simulink model "P4_car"  (R2023b)
settings: Solver=VariableStepAuto  StartTime=0.0  StopTime=201  RelTol=1e-3
values from neighbouring files (symbols this model uses):
  rps2rpm = 60/(2*pi())    [P4init.m]
  track_waypoints = [transpose(track_x), transpose(track_y)]    [genTrack.m]
undefined symbols (not defined in the file or in its folder): batData, carData, motorData
libraries: slpidlib x2
settings Model: Creator=dxego  LastModifiedBy=kami2

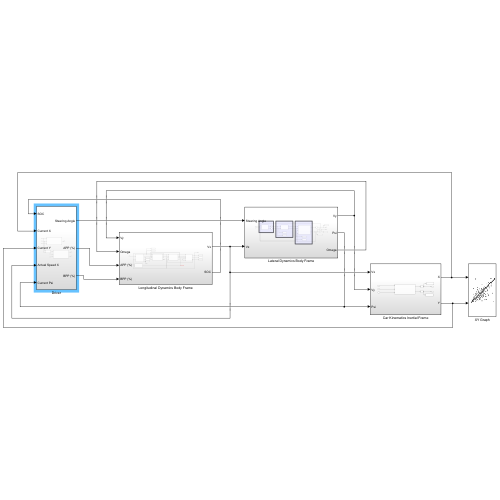
[thumbnail: Simulink's stored preview of the top-level diagram]
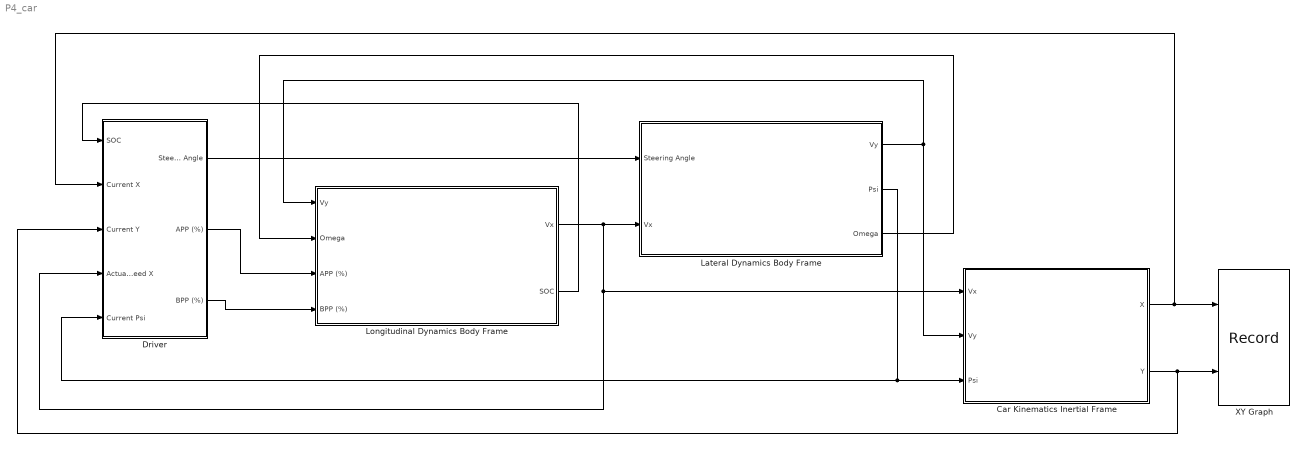
== system P4_car ==
  Car Kinematics Inertial Frame : Subsystem
  Driver : Subsystem
  Lateral Dynamics Body Frame : Subsystem
  Longitudinal Dynamics Body Frame : Subsystem
  XY Graph : Record  FileSettingsInternal="{\"entries\":[{\"content\":{\"excelSettings\":{\"content\":{},\"type\":\"Streamout.ExcelSettings\"}},\"type\":\"Streamout.FileSettingStorage\",\"uuid\":\"\"}],\"packageUris\":[\"http:\\/\\/schema.mathworks.com\\/mf0\\/streamout_blocks\\/R2020a\"],\"version\":\"1.0\"}"  Layout=[1 1]  SignalsInternal="{\"entries\":[{\"content\":{\"signals\":[{\"content\":{\"blockPath\":[],\"dimensions\":[1],\"domain\":\"\",\"lineColor\":\"#ff6929\",\"port\":1,\"sid\":[\"\"],\"signalID\":1460,\"signalName\":\"Car Kinematics Inertial Frame:1\"},\"type\":\"RecordBlkView.Signal\",\"uuid\":\"\"},{\"content\":{\"blockPath\":[],\"dimensions\":[1],\"domain\":\"\",\"lineColor\":\"#b746ff\",\"port\":2,\"sid\":[\"\"],\"signalID\":1464,\"signalName\":\"Car Kinematics Inertial Frame:2\"},\"type\":\"RecordBlkView.Signal\",\"uuid\":\"\"}]},\"type\":\"RecordBlkView.InputSignals\",\"uuid\":\"\"}],\"packageUris\":[\"http:\\/\\/schema.mathworks.com\\/mf0\\/streamout_blocks\\/R2020a\"],\"version\":\"1.0\"}"  VisualizationBindings="{\"xyplotplugin\":{\"info\":[{\"series\":[],\"subplotID\":1}]}}"  CompatibilityTag=XY  st=-1
  wires:
  Longitudinal Dynamics Body Frame/1(Vx) -> Driver/4(Actual Speed X), Car Kinematics Inertial Frame/1(Vx), Lateral Dynamics Body Frame/2(Vx)
  Lateral Dynamics Body Frame/1(Vy) -> Longitudinal Dynamics Body Frame/1(Vy), Car Kinematics Inertial Frame/2(Vy)
  Lateral Dynamics Body Frame/3(Omega) -> Longitudinal Dynamics Body Frame/2(Omega)
  Lateral Dynamics Body Frame/2(Psi) -> Car Kinematics Inertial Frame/3(Psi), Driver/5(Current Psi)
  Car Kinematics Inertial Frame/1(X) -> Driver/2(Current X), XY Graph/1
  Car Kinematics Inertial Frame/2(Y) -> XY Graph/2, Driver/3(Current Y)
  Driver/1(Steering Angle) -> Lateral Dynamics Body Frame/1(Steering Angle)
  Driver/2(APP (%)) -> Longitudinal Dynamics Body Frame/3(APP (%))
  Driver/3(BPP (%)) -> Longitudinal Dynamics Body Frame/4(BPP (%))
  Longitudinal Dynamics Body Frame/2(SOC) -> Driver/1(SOC)

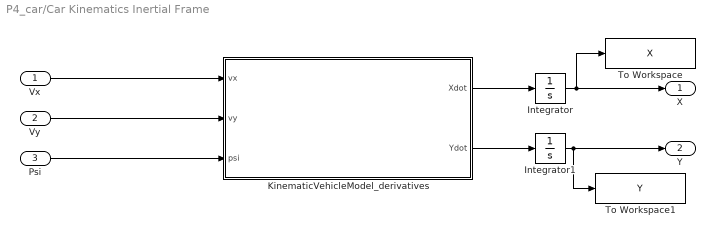
== system P4_car/Car Kinematics Inertial Frame ==
  Vx : Inport
  Vy : Inport  Port=2
  Psi : Inport  Port=3
  Integrator : Integrator  InitialCondition=carData.init.X0
  Integrator1 : Integrator  InitialCondition=carData.init.Y0
  KinematicVehicleModel_derivatives : MATLAB Function  TreatAsAtomicUnit=on  mask{obj=carData}
      mask prompts: obj "obj structure"
  To Workspace : ToWorkspace  VariableName=X  SaveFormat=Timeseries  SampleTime=-1
  To Workspace1 : ToWorkspace  VariableName=Y  SaveFormat=Timeseries  SampleTime=-1
  X : Outport
  Y : Outport  Port=2
  wires:
  KinematicVehicleModel_derivatives/1(Xdot) -> Integrator/1
  KinematicVehicleModel_derivatives/2(Ydot) -> Integrator1/1
  Integrator/1 -> To Workspace/1, X/1
  Integrator1/1 -> To Workspace1/1, Y/1
  Vx/1 -> KinematicVehicleModel_derivatives/1(vx)
  Vy/1 -> KinematicVehicleModel_derivatives/2(vy)
  Psi/1 -> KinematicVehicleModel_derivatives/3(psi)

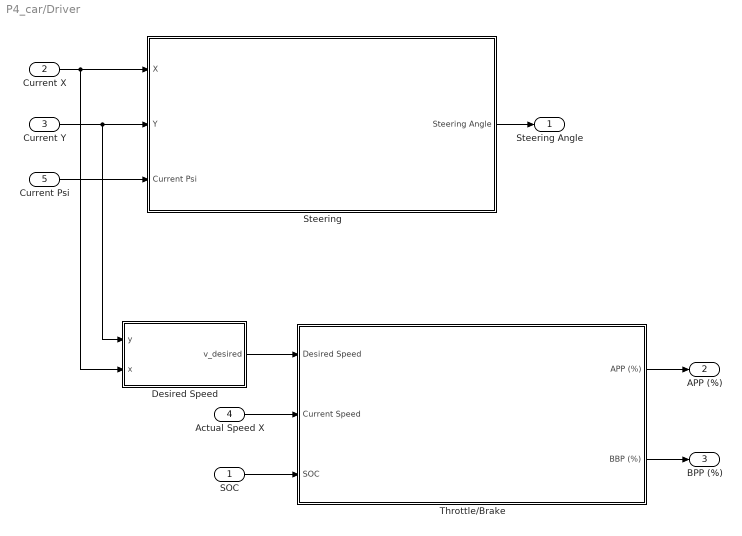
== system P4_car/Driver ==
  SOC : Inport
  Current X : Inport  Port=2
  Current Y : Inport  Port=3
  Actual Speed X : Inport  Port=4
  Current Psi : Inport  Port=5
  Desired Speed : MATLAB Function  TreatAsAtomicUnit=on
  Steering : Subsystem
  Throttle/Brake : Subsystem
  Steering Angle : Outport
  APP (%) : Outport  Port=2
  BPP (%) : Outport  Port=3
  wires:
  Current X/1 -> Desired Speed/2(x), Steering/1(X)
  Current Y/1 -> Steering/2(Y), Desired Speed/1(y)
  SOC/1 -> Throttle/Brake/3(SOC)
  Actual Speed X/1 -> Throttle/Brake/2(Current Speed)
  Throttle/Brake/1(APP (%)) -> APP (%)/1
  Throttle/Brake/2(BBP (%)) -> BPP (%)/1
  Steering/1(Steering Angle) -> Steering Angle/1
  Current Psi/1 -> Steering/3(Current Psi)
  Desired Speed/1(v_desired) -> Throttle/Brake/1(Desired Speed)

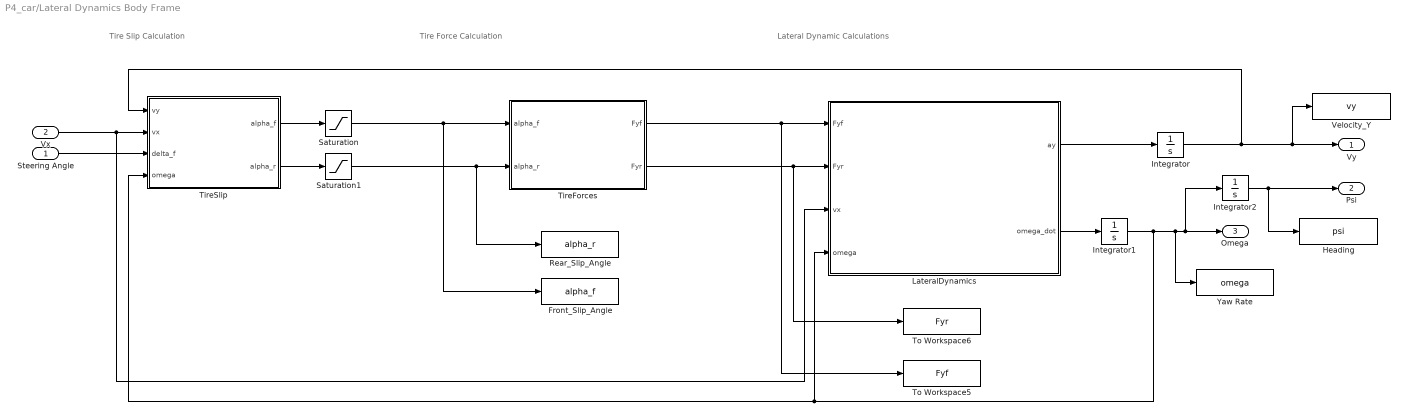
== system P4_car/Lateral Dynamics Body Frame ==
  note: Tire Slip Calculation
  note: Tire Force Calculation
  note: Lateral Dynamic Calculations
  Steering Angle : Inport
  Vx : Inport  Port=2
  Front_Slip_Angle : ToWorkspace  VariableName=alpha_f  SaveFormat=Timeseries  SampleTime=-1
  Heading : ToWorkspace  VariableName=psi  SaveFormat=Timeseries  SampleTime=-1
  Integrator : Integrator  InitialCondition=carData.init.vy0
  Integrator1 : Integrator  InitialCondition=carData.init.omega0
  Integrator2 : Integrator  InitialCondition=carData.init.psi0
  LateralDynamics : MATLAB Function  TreatAsAtomicUnit=on  mask{obj=carData}
      mask prompts: obj "obj structure"
  Rear_Slip_Angle : ToWorkspace  VariableName=alpha_r  SaveFormat=Timeseries  SampleTime=-1
  Saturation : Saturate  UpperLimit=carData.maxAlpha  LowerLimit=-carData.maxAlpha
  Saturation1 : Saturate  UpperLimit=carData.maxAlpha  LowerLimit=-carData.maxAlpha
  TireForces : MATLAB Function  TreatAsAtomicUnit=on  mask{obj=carData}
      mask prompts: obj "obj structure"
  TireSlip : MATLAB Function  TreatAsAtomicUnit=on  mask{obj=carData}
      mask prompts: obj "obj structure"
  To Workspace5 : ToWorkspace  VariableName=Fyf  SaveFormat=Timeseries  SampleTime=-1
  To Workspace6 : ToWorkspace  VariableName=Fyr  SaveFormat=Timeseries  SampleTime=-1
  Velocity_Y : ToWorkspace  VariableName=vy  SaveFormat=Timeseries  SampleTime=-1
  Yaw Rate : ToWorkspace  VariableName=omega  SaveFormat=Timeseries  SampleTime=-1
  Vy : Outport
  Psi : Outport  Port=2
  Omega : Outport  Port=3
  wires:
  LateralDynamics/1(ay) -> Integrator/1
  Integrator/1 -> Vy/1, Velocity_Y/1, TireSlip/1(vy)
  LateralDynamics/2(omega_dot) -> Integrator1/1
  Integrator1/1 -> Integrator2/1, Omega/1, Yaw Rate/1, LateralDynamics/4(omega), TireSlip/4(omega)
  TireSlip/1(alpha_f) -> Saturation/1
  TireSlip/2(alpha_r) -> Saturation1/1
  TireForces/1(Fyf) -> LateralDynamics/1(Fyf), To Workspace5/1
  TireForces/2(Fyr) -> LateralDynamics/2(Fyr), To Workspace6/1
  Saturation/1 -> TireForces/1(alpha_f), Front_Slip_Angle/1
  Saturation1/1 -> TireForces/2(alpha_r), Rear_Slip_Angle/1
  Vx/1 -> TireSlip/2(vx), LateralDynamics/3(vx)
  Steering Angle/1 -> TireSlip/3(delta_f)
  Integrator2/1 -> Heading/1, Psi/1

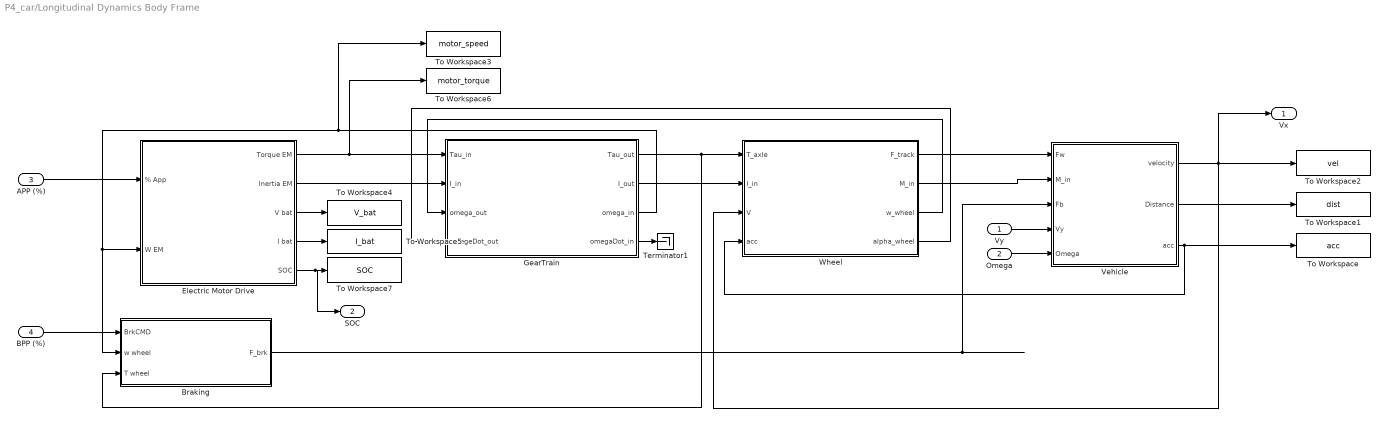
== system P4_car/Longitudinal Dynamics Body Frame ==
  Vy : Inport
  Omega : Inport  Port=2
  APP (%) : Inport  Port=3
  BPP (%) : Inport  Port=4
  Braking : Subsystem
  Electric Motor Drive : Subsystem
  GearTrain : Subsystem
  Terminator1 : Terminator
  To Workspace : ToWorkspace  VariableName=acc  SaveFormat=Timeseries  SampleTime=-1
  To Workspace1 : ToWorkspace  VariableName=dist  SaveFormat=Timeseries  SampleTime=-1
  To Workspace2 : ToWorkspace  VariableName=vel  SaveFormat=Timeseries  SampleTime=-1
  To Workspace3 : ToWorkspace  VariableName=motor_speed  SaveFormat=Timeseries  SampleTime=-1
  To Workspace4 : ToWorkspace  VariableName=V_bat  SaveFormat=Timeseries  SampleTime=-1
  To Workspace5 : ToWorkspace  VariableName=I_bat  SaveFormat=Timeseries  SampleTime=-1
  To Workspace6 : ToWorkspace  VariableName=motor_torque  SaveFormat=Timeseries  SampleTime=-1
  To Workspace7 : ToWorkspace  VariableName=SOC  SaveFormat=Timeseries  SampleTime=-1
  Vehicle : Subsystem
  "Wheel " : Subsystem
  Vx : Outport
  SOC : Outport  Port=2
  wires:
  "Wheel "/2(M_in) -> Vehicle/2("M_in ")
  Electric Motor Drive/2(Inertia EM) -> GearTrain/2(I_in)
  GearTrain/4(omegaDot_in) -> Terminator1/1
  Electric Motor Drive/3(V bat) -> To Workspace4/1
  Vehicle/2("Distance ") -> To Workspace1/1
  Electric Motor Drive/1(Torque EM) -> To Workspace6/1, GearTrain/1(Tau_in)
  Vehicle/3(acc) -> "Wheel "/4(acc), To Workspace/1
  Electric Motor Drive/4(I bat) -> To Workspace5/1
  "Wheel "/3(w_wheel) -> GearTrain/3(omega_out)
  GearTrain/3(omega_in) -> To Workspace3/1, Electric Motor Drive/2(W EM), Braking/2("w wheel ")
  Vehicle/1("velocity ") -> Vx/1, To Workspace2/1, "Wheel "/3(V)
  "Wheel "/4(alpha_wheel) -> GearTrain/4(omegeDot_out)
  Braking/1("F_brk ") -> Vehicle/3("Fb ")
  GearTrain/1(Tau_out) -> Braking/3(T wheel), "Wheel "/1(T_axle)
  "Wheel "/1(F_track) -> Vehicle/1("Fw ")
  GearTrain/2(I_out) -> "Wheel "/2(I_in)
  Electric Motor Drive/5(SOC) -> SOC/1, To Workspace7/1
  APP (%)/1 -> Electric Motor Drive/1(% App)
  BPP (%)/1 -> Braking/1("BrkCMD ")
  Vy/1 -> Vehicle/4(Vy)
  Omega/1 -> Vehicle/5(Omega)

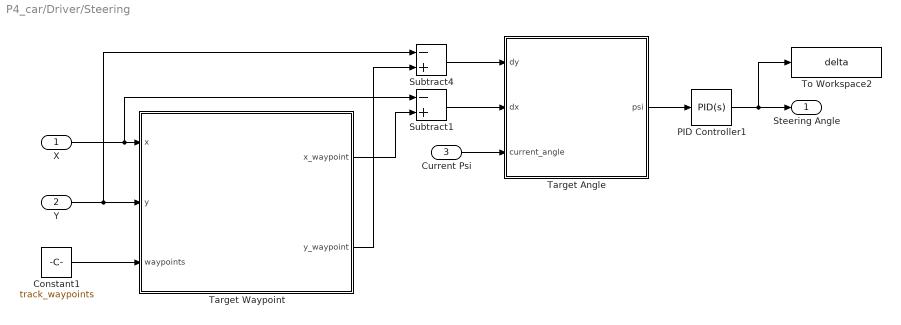
== system P4_car/Driver/Steering ==
  X : Inport
  Y : Inport  Port=2
  Current Psi : Inport  Port=3
  Constant1 : Constant  Value=track_waypoints
  PID Controller1 : slpidlib/PID Controller  Controller=PID  Form=Parallel  TimeDomain=Continuous-time  UseExternalTs=off  SampleTime=-1  IntegratorMethod=Forward Euler  FilterMethod=Forward Euler  ControllerParametersSource=internal  P=0.5  I=0  UseKiTs=off  D=0  N=100  UseFilter=on  TunerSelectOption=Transfer Function Based (PID Tuner App)  InitialConditionSource=internal  InitialConditionForIntegrator=0  InitialConditionForFilter=0  DifferentiatorICPrevScaledInput=0  ExternalReset=none  TrackingMode=off  Kt=1  LimitOutput=off  SatLimitsSource=internal  UpperSaturationLimit=inf  LowerSaturationLimit=-inf  LinearizeAsGain=on  AntiWindupMode=none  Kb=1  LimitIntegrator=off  UpperIntegratorSaturationLimit=inf  LowerIntegratorSaturationLimit=-inf  POutMin=[]  POutMax=[]  IOutMin=[]  IOutMax=[]  DOutMin=[]  DOutMax=[]  NOutMin=[]  NOutMax=[]  SumOutMin=[]  SumOutMax=[]  SaturationOutMin=[]  SaturationOutMax=[]  PParamMin=[]  PParamMax=[]  IParamMin=[]  IParamMax=[]  DParamMin=[]  DParamMax=[]  NParamMin=[]  NParamMax=[]  KbParamMin=[]  KbParamMax=[]  KtParamMin=[]  KtParamMax=[]  KbOutMin=[]  KbOutMax=[]  KtOutMin=[]  KtOutMax=[]  IntegratorOutMin=[]  IntegratorOutMax=[]  FilterOutMin=[]  FilterOutMax=[]  SumI1OutMin=[]  SumI1OutMax=[]  SumI2OutMin=[]  SumI2OutMax=[]  SumI3OutMin=[]  SumI3OutMax=[]  SumI4OutMin=[]  SumI4OutMax=[]  SumDOutMin=[]  SumDOutMax=[]  DifferentiatorOutMin=[]  DifferentiatorOutMax=[]  FilterDiffOutCoefMin=[]  FilterDiffOutCoefMax=[]  ReciprocalOutMin=[]  ReciprocalOutMax=[]  SumDenOutMin=[]  SumDenOutMax=[]  SumNumOutMin=[]  SumNumOutMax=[]  DivideOutMin=[]  DivideOutMax=[]  UdiffTsProdOutMin=[]  UdiffTsProdOutMax=[]  NTsProdOutMin=[]  NTsProdOutMax=[]  UintegralTsProdOutMin=[]  UintegralTsProdOutMax=[]  UngainTsProdOutMin=[]  UngainTsProdOutMax=[]  ClampingZeroOutDataTypeStr=Inherit: Inherit via back propagation  ClampingZeroOutMin=[]  ClampingZeroOutMax=[]  FilterDenConstantOutDataTypeStr=Inherit: Inherit via back propagation  FilterDenConstantOutMin=[]  FilterDenConstantOutMax=[]  PCopyOutDataTypeStr=Inherit: Inherit via back propagation  PCopyOutMin=[]  PCopyOutMax=[]  NCopyOutDataTypeStr=Inherit: Inherit via back propagation  NCopyOutMin=[]  NCopyOutMax=[]  IntegratorContinuousStateAttributes=''  IntegratorStateMustResolveToSignalObject=off  IntegratorRTWStateStorageClass=Auto  FilterContinuousStateAttributes=''  FilterStateMustResolveToSignalObject=off  FilterRTWStateStorageClass=Auto  ParallelPVariant=InternalParameters  IdealPVariant=Disabled  IVariant=InternalParameters  DVariant=InternalParameters  IntegratorVariant=Continuous  SatVariant=Disabled  AWVariant=Passthrough  PCopyVariant=Disabled  TRVariant=Disabled  FdbkBlocksVariant=Forward  IdealPFdbkVariant=Disabled  SatFdbkVariant=Disabled  DerivativeFilterVariant=ContFilter  NVariant=InternalParameters  NCopyVariant=Disabled  FilterICVariant=InternalICsFilter  IntegratorICVariant=InternalICs  ExternalResetVariant=Disabled  TRSumVariant=Passthrough  SumFdbkVariant=Disabled  SumVariant=Sum_PID  TsampFilterVariant=InternalTs  TsampNgainVariant=Passthrough  TsampIntegralVariant=Disabled_SignalSpec  ExternalSaturationOutDataTypeStr=Inherit: Same as second input
  Subtract1 : Sum  Inputs=-+
  Subtract4 : Sum  Inputs=-+
  Target Angle : MATLAB Function  TreatAsAtomicUnit=on
  Target Waypoint : MATLAB Function  TreatAsAtomicUnit=on
  To Workspace2 : ToWorkspace  VariableName=delta  SaveFormat=Timeseries  SampleTime=-1
  Steering Angle : Outport
  wires:
  Constant1/1 -> Target Waypoint/3(waypoints)
  Target Waypoint/2(y_waypoint) -> Subtract4/2
  Y/1 -> Subtract4/1, Target Waypoint/2(y)
  X/1 -> Target Waypoint/1(x), Subtract1/1
  Subtract1/1 -> Target Angle/2(dx)
  Target Angle/1(psi) -> PID Controller1/1
  Current Psi/1 -> Target Angle/3(current_angle)
  Target Waypoint/1(x_waypoint) -> Subtract1/2
  Subtract4/1 -> Target Angle/1(dy)
  PID Controller1/1 -> To Workspace2/1, Steering Angle/1

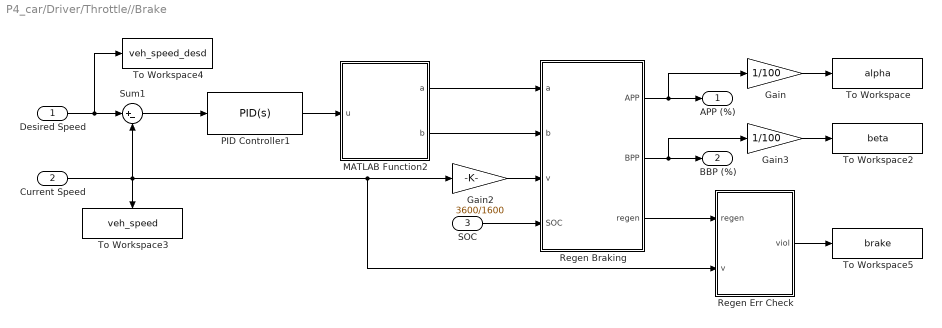
== system P4_car/Driver/Throttle//Brake ==
  Desired Speed : Inport
  Current Speed : Inport  Port=2
  SOC : Inport  Port=3
  Gain : Gain  Gain=1/100
  Gain2 : Gain  Gain=3600/1600
  Gain3 : Gain  Gain=1/100
  MATLAB Function2 : MATLAB Function  TreatAsAtomicUnit=on
  PID Controller1 : slpidlib/PID Controller  Controller=PID  Form=Parallel  TimeDomain=Continuous-time  UseExternalTs=off  SampleTime=-1  IntegratorMethod=Forward Euler  FilterMethod=Forward Euler  ControllerParametersSource=internal  P=.5  I=0  UseKiTs=off  D=0  N=100  UseFilter=on  TunerSelectOption=Transfer Function Based (PID Tuner App)  InitialConditionSource=internal  InitialConditionForIntegrator=0  InitialConditionForFilter=0  DifferentiatorICPrevScaledInput=0  ExternalReset=none  TrackingMode=off  Kt=1  LimitOutput=on  SatLimitsSource=internal  UpperSaturationLimit=1  LowerSaturationLimit=-1  LinearizeAsGain=off  AntiWindupMode=none  Kb=1  LimitIntegrator=off  UpperIntegratorSaturationLimit=inf  LowerIntegratorSaturationLimit=-inf  POutMin=[]  POutMax=[]  IOutMin=[]  IOutMax=[]  DOutMin=[]  DOutMax=[]  NOutMin=[]  NOutMax=[]  SumOutMin=[]  SumOutMax=[]  SaturationOutMin=[]  SaturationOutMax=[]  PParamMin=[]  PParamMax=[]  IParamMin=[]  IParamMax=[]  DParamMin=[]  DParamMax=[]  NParamMin=[]  NParamMax=[]  KbParamMin=[]  KbParamMax=[]  KtParamMin=[]  KtParamMax=[]  KbOutMin=[]  KbOutMax=[]  KtOutMin=[]  KtOutMax=[]  IntegratorOutMin=[]  IntegratorOutMax=[]  FilterOutMin=[]  FilterOutMax=[]  SumI1OutMin=[]  SumI1OutMax=[]  SumI2OutMin=[]  SumI2OutMax=[]  SumI3OutMin=[]  SumI3OutMax=[]  SumI4OutMin=[]  SumI4OutMax=[]  SumDOutMin=[]  SumDOutMax=[]  DifferentiatorOutMin=[]  DifferentiatorOutMax=[]  FilterDiffOutCoefMin=[]  FilterDiffOutCoefMax=[]  ReciprocalOutMin=[]  ReciprocalOutMax=[]  SumDenOutMin=[]  SumDenOutMax=[]  SumNumOutMin=[]  SumNumOutMax=[]  DivideOutMin=[]  DivideOutMax=[]  UdiffTsProdOutMin=[]  UdiffTsProdOutMax=[]  NTsProdOutMin=[]  NTsProdOutMax=[]  UintegralTsProdOutMin=[]  UintegralTsProdOutMax=[]  UngainTsProdOutMin=[]  UngainTsProdOutMax=[]  ClampingZeroOutDataTypeStr=Inherit: Inherit via back propagation  ClampingZeroOutMin=[]  ClampingZeroOutMax=[]  FilterDenConstantOutDataTypeStr=Inherit: Inherit via back propagation  FilterDenConstantOutMin=[]  FilterDenConstantOutMax=[]  PCopyOutDataTypeStr=Inherit: Inherit via back propagation  PCopyOutMin=[]  PCopyOutMax=[]  NCopyOutDataTypeStr=Inherit: Inherit via back propagation  NCopyOutMin=[]  NCopyOutMax=[]  IntegratorContinuousStateAttributes=''  IntegratorStateMustResolveToSignalObject=off  IntegratorRTWStateStorageClass=Auto  FilterContinuousStateAttributes=''  FilterStateMustResolveToSignalObject=off  FilterRTWStateStorageClass=Auto  ParallelPVariant=InternalParameters  IdealPVariant=Disabled  IVariant=InternalParameters  DVariant=InternalParameters  IntegratorVariant=Continuous  SatVariant=Enabled  AWVariant=Passthrough  PCopyVariant=Disabled  TRVariant=Disabled  FdbkBlocksVariant=Forward  IdealPFdbkVariant=Disabled  SatFdbkVariant=Disabled  DerivativeFilterVariant=ContFilter  NVariant=InternalParameters  NCopyVariant=Disabled  FilterICVariant=InternalICsFilter  IntegratorICVariant=InternalICs  ExternalResetVariant=Disabled  TRSumVariant=Passthrough  SumFdbkVariant=Disabled  SumVariant=Sum_PID  TsampFilterVariant=InternalTs  TsampNgainVariant=Passthrough  TsampIntegralVariant=Disabled_SignalSpec  ExternalSaturationOutDataTypeStr=Inherit: Same as second input
  Regen Braking : MATLAB Function  TreatAsAtomicUnit=on
  Regen Err Check : MATLAB Function  TreatAsAtomicUnit=on
  Sum1 : Sum  Inputs=|+-
  To Workspace : ToWorkspace  VariableName=alpha  SaveFormat=Timeseries  SampleTime=-1
  To Workspace2 : ToWorkspace  VariableName=beta  SaveFormat=Timeseries  SampleTime=-1
  To Workspace3 : ToWorkspace  VariableName=veh_speed  SaveFormat=Timeseries  SampleTime=-1
  To Workspace4 : ToWorkspace  VariableName=veh_speed_desd  SaveFormat=Timeseries  SampleTime=-1
  To Workspace5 : ToWorkspace  VariableName=brake  SaveFormat=Timeseries  SampleTime=-1
  APP (%) : Outport
  BBP (%) : Outport  Port=2
  wires:
  PID Controller1/1 -> MATLAB Function2/1(u)
  MATLAB Function2/2(b) -> Regen Braking/2(b)
  Regen Braking/3(regen) -> Regen Err Check/1(regen)
  Regen Braking/2(BPP) -> Gain3/1, BBP (%)/1
  Regen Err Check/1(viol) -> To Workspace5/1
  SOC/1 -> Regen Braking/4(SOC)
  Desired Speed/1 -> To Workspace4/1, Sum1/1
  MATLAB Function2/1(a) -> Regen Braking/1(a)
  Sum1/1 -> PID Controller1/1
  Current Speed/1 -> To Workspace3/1, Sum1/2, Regen Err Check/2(v), Gain2/1
  Gain2/1 -> Regen Braking/3(v)
  Regen Braking/1(APP) -> Gain/1, APP (%)/1
  Gain/1 -> To Workspace/1
  Gain3/1 -> To Workspace2/1

== system P4_car/Longitudinal Dynamics Body Frame/Braking ==
  "BrkCMD " : Inport
  "w wheel " : Inport  Port=2
  T wheel : Inport  Port=3
  Constant : Constant  Value=15000
  MATLAB Function : MATLAB Function  TreatAsAtomicUnit=on
  Terminator : Terminator
  To Workspace6 : ToWorkspace  VariableName=brake_torque  SaveFormat=Timeseries  SampleTime=-1
  TorqueToForce : Gain  Gain=1/carData.r
  "F_brk " : Outport  VectorParamsAs1DForOutWhenUnconnected=off
  wires:
  "BrkCMD "/1 -> MATLAB Function/1(brakePer)
  MATLAB Function/1(y) -> To Workspace6/1, TorqueToForce/1
  "w wheel "/1 -> MATLAB Function/3(Ww)
  TorqueToForce/1 -> "F_brk "/1
  Constant/1 -> MATLAB Function/2(Tmax)
  T wheel/1 -> Terminator/1

== system P4_car/Longitudinal Dynamics Body Frame/Electric Motor Drive ==
  % App : Inport
  W EM : Inport  Port=2
  Bat : Subsystem
  EM : Subsystem
  Torque EM : Outport
  Inertia EM : Outport  Port=2
  V bat : Outport  Port=3
  I bat : Outport  Port=4
  SOC : Outport  Port=5
  wires:
  % App/1 -> EM/2(% app)
  W EM/1 -> EM/3(motor speed (rad/s))
  EM/1(I bus) -> I bat/1, Bat/1(I bat)
  EM/2(Motor Torque (Nm)) -> Torque EM/1
  EM/3(I Motor) -> Inertia EM/1
  Bat/2(SOC) -> SOC/1
  Bat/1(V bat) -> EM/1(Bus V), V bat/1

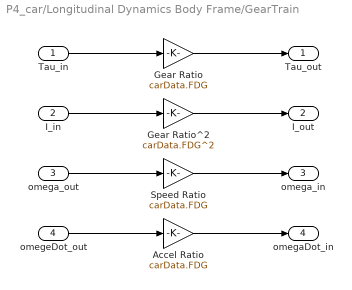
== system P4_car/Longitudinal Dynamics Body Frame/GearTrain ==
  Tau_in : Inport
  I_in : Inport  Port=2
  omega_out : Inport  Port=3
  omegeDot_out : Inport  Port=4
  Accel Ratio : Gain  Gain=carData.FDG
  Gear Ratio : Gain  Gain=carData.FDG
  Gear Ratio^2 : Gain  Gain=carData.FDG^2
  Speed Ratio : Gain  Gain=carData.FDG
  Tau_out : Outport
  I_out : Outport  Port=2
  omega_in : Outport  Port=3
  omegaDot_in : Outport  Port=4
  wires:
  Tau_in/1 -> Gear Ratio/1
  Gear Ratio/1 -> Tau_out/1
  Gear Ratio^2/1 -> I_out/1
  I_in/1 -> Gear Ratio^2/1
  Speed Ratio/1 -> omega_in/1
  omega_out/1 -> Speed Ratio/1
  Accel Ratio/1 -> omegaDot_in/1
  omegeDot_out/1 -> Accel Ratio/1

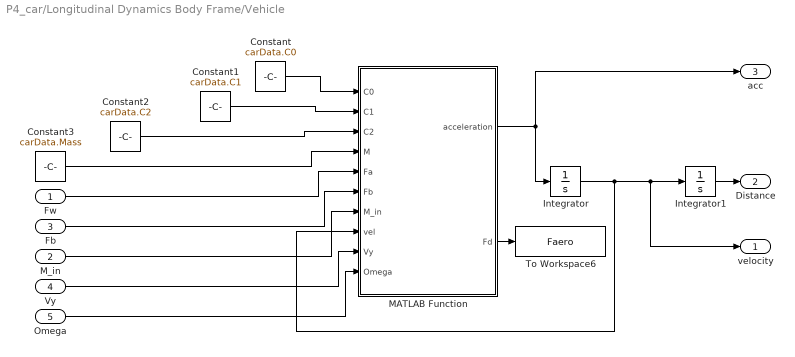
== system P4_car/Longitudinal Dynamics Body Frame/Vehicle ==
  "Fw " : Inport
  "M_in " : Inport  Port=2
  "Fb " : Inport  Port=3
  Vy : Inport  Port=4
  Omega : Inport  Port=5
  Constant : Constant  Value=carData.C0
  Constant1 : Constant  Value=carData.C1
  Constant2 : Constant  Value=carData.C2
  Constant3 : Constant  Value=carData.Mass
  Integrator : Integrator  LimitOutput=on  LowerSaturationLimit=0
  Integrator1 : Integrator
  MATLAB Function : MATLAB Function  TreatAsAtomicUnit=on
  To Workspace6 : ToWorkspace  VariableName=Faero  SaveFormat=Timeseries  SampleTime=-1
  "velocity " : Outport  VectorParamsAs1DForOutWhenUnconnected=off
  "Distance " : Outport  Port=2  VectorParamsAs1DForOutWhenUnconnected=off
  acc : Outport  Port=3
  wires:
  Constant1/1 -> MATLAB Function/2(C1)
  Constant/1 -> MATLAB Function/1(C0)
  MATLAB Function/1(acceleration) -> Integrator/1, acc/1
  Constant2/1 -> MATLAB Function/3(C2)
  Constant3/1 -> MATLAB Function/4(M)
  "Fw "/1 -> MATLAB Function/5(Fa)
  "Fb "/1 -> MATLAB Function/6(Fb)
  Integrator/1 -> MATLAB Function/8(vel), "velocity "/1, Integrator1/1
  Integrator1/1 -> "Distance "/1
  "M_in "/1 -> MATLAB Function/7(M_in)
  Vy/1 -> MATLAB Function/9(Vy)
  Omega/1 -> MATLAB Function/10(Omega)
  MATLAB Function/2(Fd) -> To Workspace6/1

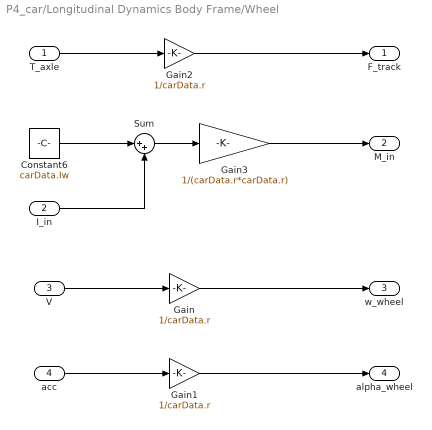
== system P4_car/Longitudinal Dynamics Body Frame/Wheel  ==
  T_axle : Inport
  I_in : Inport  Port=2
  V : Inport  Port=3
  acc : Inport  Port=4
  Constant6 : Constant  Value=carData.Iw
  Gain : Gain  Gain=1/carData.r
  Gain1 : Gain  Gain=1/carData.r
  Gain2 : Gain  Gain=1/carData.r
  Gain3 : Gain  Gain=1/(carData.r*carData.r)
  Sum : Sum  Inputs=|++
  F_track : Outport
  M_in : Outport  Port=2
  w_wheel : Outport  Port=3
  alpha_wheel : Outport  Port=4
  wires:
  Gain/1 -> w_wheel/1
  V/1 -> Gain/1
  acc/1 -> Gain1/1
  Gain1/1 -> alpha_wheel/1
  T_axle/1 -> Gain2/1
  Gain2/1 -> F_track/1
  Gain3/1 -> M_in/1
  Constant6/1 -> Sum/1
  I_in/1 -> Sum/2
  Sum/1 -> Gain3/1

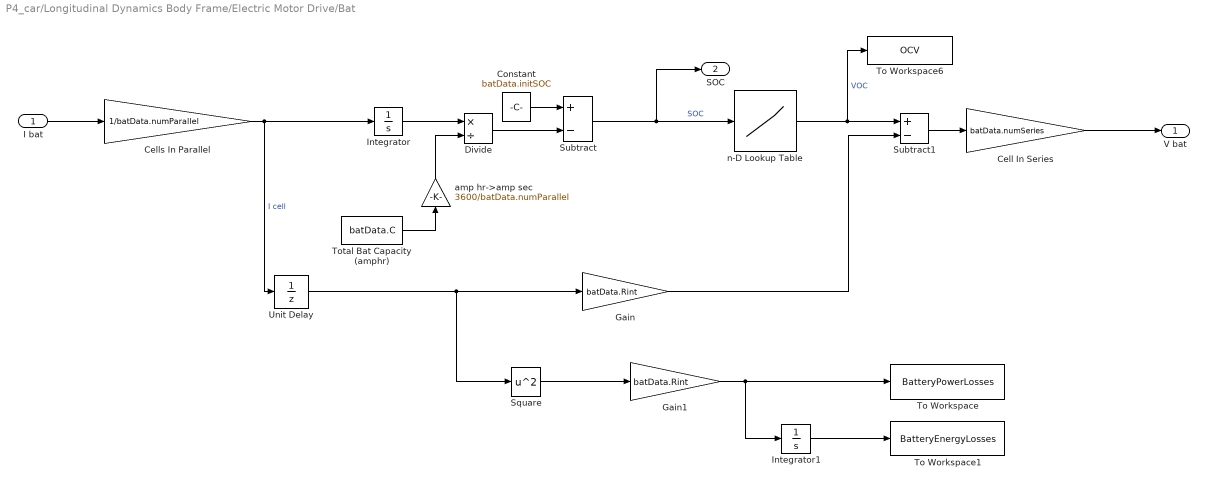
== system P4_car/Longitudinal Dynamics Body Frame/Electric Motor Drive/Bat ==
  I bat : Inport
  Cell In Series : Gain  Gain=batData.numSeries
  Cells In Parallel : Gain  Gain=1/batData.numParallel
  Constant : Constant  Value=batData.initSOC
  Divide : Product  Inputs=*/
  Gain : Gain  Gain=batData.Rint
  Gain1 : Gain  Gain=batData.Rint
  Integrator : Integrator
  Integrator1 : Integrator
  Square : Math  Operator=square
  Subtract : Sum  Inputs=+-
  Subtract1 : Sum  Inputs=+-
  To Workspace : ToWorkspace  VariableName=BatteryPowerLosses  SaveFormat=Timeseries  SampleTime=-1
  To Workspace1 : ToWorkspace  VariableName=BatteryEnergyLosses  SaveFormat=Timeseries  SampleTime=-1
  To Workspace6 : ToWorkspace  VariableName=OCV  SaveFormat=Timeseries  SampleTime=-1
  Total Bat Capacity (amphr) : Constant  Value=batData.C
  Unit Delay : UnitDelay  SampleTime=-1  HasFrameUpgradeWarning=on
  amp hr->amp sec : Gain  Gain=3600/batData.numParallel
  n-D Lookup Table : Lookup_n-D  NumberOfTableDimensions=1  BreakpointsForDimension1=batData.SOC  BreakpointsForDimension3=[5, 7]  Table=batData.OCV  InternalRulePriority=Speed  RndMeth=Simplest
  V bat : Outport
  SOC : Outport  Port=2
  wires:
  Cells In Parallel/1 -> Unit Delay/1, Integrator/1  "I cell"
  I bat/1 -> Cells In Parallel/1
  Integrator/1 -> Divide/1
  Total Bat Capacity (amphr)/1 -> amp hr->amp sec/1
  amp hr->amp sec/1 -> Divide/2
  Divide/1 -> Subtract/2
  Constant/1 -> Subtract/1
  Subtract/1 -> SOC/1, n-D Lookup Table/1  "SOC"
  n-D Lookup Table/1 -> To Workspace6/1, Subtract1/1  "VOC"
  Unit Delay/1 -> Square/1, Gain/1
  Gain/1 -> Subtract1/2
  Subtract1/1 -> Cell In Series/1
  Cell In Series/1 -> V bat/1
  Square/1 -> Gain1/1
  Gain1/1 -> Integrator1/1, To Workspace/1
  Integrator1/1 -> To Workspace1/1

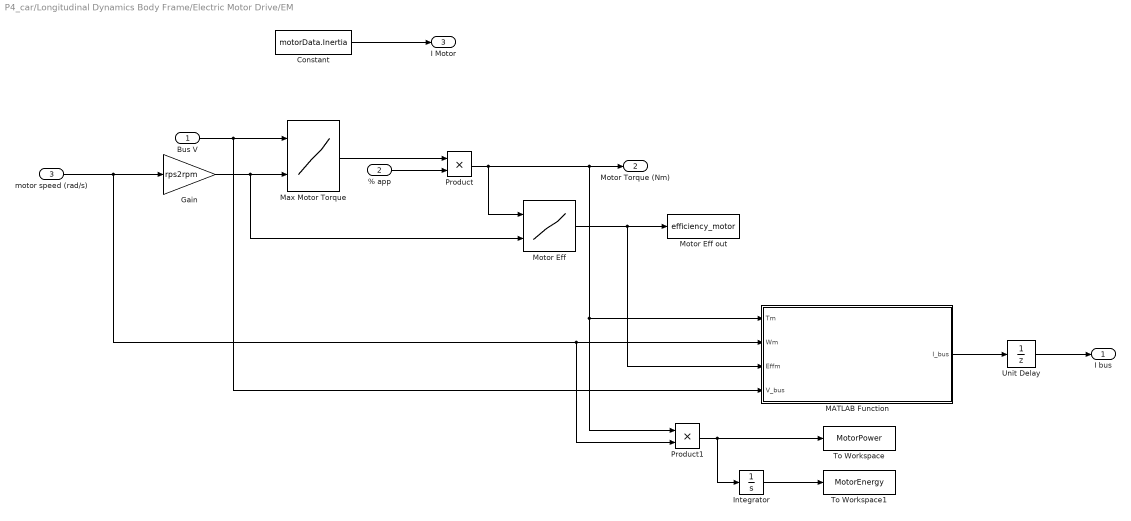
== system P4_car/Longitudinal Dynamics Body Frame/Electric Motor Drive/EM ==
  Bus V : Inport
  % app : Inport  Port=2
  motor speed (rad/s) : Inport  Port=3
  Constant : Constant  Value=motorData.Inertia
  Gain : Gain  Gain=rps2rpm
  Integrator : Integrator
  MATLAB Function : MATLAB Function  TreatAsAtomicUnit=on
  Max Motor Torque : Lookup_n-D  BreakpointsForDimension1=motorData.vbus  BreakpointsForDimension2=motorData.rpm  BreakpointsForDimension3=[5, 7]  Table=motorData.maxtorque  InternalRulePriority=Speed  RndMeth=Simplest
      settings: InputPortMap=u0,u1
  Motor Eff : Lookup_n-D  BreakpointsForDimension1=motorData.eta_torque  BreakpointsForDimension2=motorData.eta_speed  BreakpointsForDimension3=[5, 7]  Table=motorData.eta_val  InternalRulePriority=Speed  RndMeth=Simplest
      settings: InputPortMap=u0,u1
  Motor Eff out : ToWorkspace  VariableName=efficiency_motor  SaveFormat=Timeseries  SampleTime=-1
  Product : Product
  Product1 : Product
  To Workspace : ToWorkspace  VariableName=MotorPower  SaveFormat=Timeseries  SampleTime=-1
  To Workspace1 : ToWorkspace  VariableName=MotorEnergy  SaveFormat=Timeseries  SampleTime=-1
  Unit Delay : UnitDelay  SampleTime=-1  HasFrameUpgradeWarning=on
  I bus : Outport
  Motor Torque (Nm) : Outport  Port=2
  I Motor : Outport  Port=3
  wires:
  motor speed (rad/s)/1 -> Product1/2, MATLAB Function/2(Wm), Gain/1
  Gain/1 -> Motor Eff/2, Max Motor Torque/2
  Bus V/1 -> Max Motor Torque/1, MATLAB Function/4(V_bus)
  Max Motor Torque/1 -> Product/1
  % app/1 -> Product/2
  Product/1 -> Motor Eff/1, Product1/1, MATLAB Function/1(Tm), Motor Torque (Nm)/1
  Motor Eff/1 -> MATLAB Function/3(Effm), Motor Eff out/1
  Constant/1 -> I Motor/1
  Product1/1 -> Integrator/1, To Workspace/1
  Integrator/1 -> To Workspace1/1
  MATLAB Function/1(I_bus) -> Unit Delay/1
  Unit Delay/1 -> I bus/1

== matlab function P4_car/Longitudinal Dynamics Body Frame/Vehicle/MATLAB Function ==
  data: C0 input; acceleration output; C1 input; C2 input; M input; Fa input; Fb input; M_in input; vel input; Vy input; Omega input; Fd output
function [acceleration, Fd] = vehicle(C0,C1,C2,M,Fa,Fb,M_in, vel, Vy, Omega)

Fd = (C0+ C1*vel + C2*(vel)^2);

acceleration = ((Fa-Fb-Fd)/(M+M_in)) + Vy*Omega;

== matlab function P4_car/Driver/Steering/Target Angle ==
  data: dy input; dx input; psi output; current_angle input
function psi = fcn(dy, dx, current_angle)

    desired_angle = atan2(dy, dx);

    if desired_angle < 0
        desired_angle = desired_angle + 2 * pi;
    end

    psi = angdiff(current_angle, desired_angle);

== matlab function P4_car/Driver/Steering/Target Waypoint ==
  data: x input; y input; waypoints input; x_waypoint output; y_waypoint output
function [x_waypoint, y_waypoint] = fcn(x, y, waypoints)

    waypoints = waypoints(1:end-1,:);
    
    % Closest Waypoint
    dist_from_waypoints = sqrt((waypoints(:,1)-x).^2+(waypoints(:,2)-y).^2);
    [~, idx] = min(dist_from_waypoints);
    
    % Look Ahead
    target_idx = idx + 3;

    if target_idx >= height(waypoints)
       target_idx = 1;
    end

    x_waypoint = waypoints(target_idx,1);
    y_waypoint = waypoints(target_idx,2);

== matlab function P4_car/Driver/Desired Speed ==
  data: y input; x input; v_desired output
function v_desired = fcn(y, x)
    
    % top straight
    if y >= 200 && x <= 900 && x >= 400
        v_desired = 26;
    % slow down and left turn
    elseif (y > 200 && x < 400) || (y < 200 && x < 0)
        v_desired = 15;
    % bottom straight
    elseif y < 200 && x <= 500 && x >= 0
        v_desired = 26;
    % slow down and right turn
    elseif (y < 200 && x > 500) || (y >= 200 && x > 900)
        v_desired = 15;
    else
        v_desired = 15;
    end

== matlab function P4_car/Lateral Dynamics Body Frame/LateralDynamics ==
  data: Fyf input; Fyr input size=1; vx input; omega input; ay output; obj parameter; omega_dot output
function [ay, omega_dot] = fcn(Fyf, Fyr, vx, omega, obj)

Fy = Fyf + Fyr;
ay = Fy / obj.Mass - omega * vx;
        
M  = Fyf * obj.lf - Fyr * obj.lr;        
omega_dot = M / obj.Inertia;        

end

== matlab function P4_car/Driver/Throttle//Brake/MATLAB Function2 ==
  data: u input; a output; b output
function [a,b] = fcn(u)

    if u>0
        acc=u;
        brk=0;
    elseif u<0
        acc=0;
        brk=-u;
    else
        acc=0;
        brk=0;
    end

    a= acc;
    b= brk;

== matlab function P4_car/Car Kinematics Inertial Frame/KinematicVehicleModel_derivatives ==
  data: vx input; vy input; psi input size=1; Xdot output; Ydot output
function [Xdot, Ydot] = fcn(vx, vy, psi)
    temp = TF(psi) * [vx;vy]; 
    Xdot = temp(1);
    Ydot = temp(2);
  
end

function y = TF(psi)
    y = [cos(psi), -sin(psi); sin(psi), cos(psi)];
end

== matlab function P4_car/Longitudinal Dynamics Body Frame/Braking/MATLAB Function ==
  data: brakePer input; Tmax input; y output; Ww input
function y = fcn(brakePer,Tmax, Ww)
%y =u*sign(v)
%y = u * v/(abs(v)+0.001);
%y = u;

% u = % brake force applied
% Tmax = max brake torque available * mu (pad friction) * gb (design
% factor)
% v = angular velocity, velocity is used bc omega/velocity will have same
% sign, which is all we are concerned about

% check for lock/unlocked
% when locked, brake torque = max brake torque
% when brakes not locked, brake torque = Tmax*u*sgn(w)
% sgn: if w<0, = -1; w=0, = 0; w>0, = 1

% non locked case
if brakePer < 1
    y = (Tmax * brakePer) * Ww/(Ww+0.001);

% locked case
else
    y = Tmax;
end

== matlab function P4_car/Driver/Throttle//Brake/Regen Err Check ==
  data: regen input; viol output; v input
function viol = violfcn(regen, v)
    speed = (3600/1600)*v;
    if speed < 5
        regen_vio = 0;
        if regen == regen_vio
            viol = 0;
        else
            viol = 1;
        end

    elseif speed == 25
        regen_vio = 0.95;
        if regen == regen_vio
            viol = 0;
        else
            viol = 1;
        end

    elseif v > 25
        regen_vio = 0.95;
        if regen == regen_vio
            viol = 0;
        else
            viol = 1;
        end
    else
        regen_vio = ((0.95/20)*speed)-0.2375;
        if regen == regen_vio
            viol = 0;
        else
            viol = 1;
        end
    end

== matlab function P4_car/Lateral Dynamics Body Frame/TireSlip ==
  data: vy input size=1; vx input; delta_f input size=1; omega input; alpha_f output; obj parameter; alpha_r output
function [alpha_f, alpha_r] = fcn(vy,  vx, delta_f, omega, obj)


if abs(vx)> obj.vx_threshold1
      alpha_f = delta_f - (vy + omega * obj.lf) / vx;
      alpha_r = - (vy - omega * obj.lr) / vx;
else
      alpha_f = 0;
      alpha_r = 0;
end



end

== matlab function P4_car/Lateral Dynamics Body Frame/TireForces ==
  data: alpha_f input; alpha_r input; Fyf output; obj parameter; Fyr output
function [Fyf, Fyr] = fcn(alpha_f, alpha_r, obj)

Fyf = min(obj.Fyfmax,obj.Calpha_f * alpha_f);
Fyr = min(obj.Fyrmax, obj.Calpha_r * alpha_r);
end

== matlab function P4_car/Driver/Throttle//Brake/Regen Braking ==
  data: a input; APP output; b input; v input; SOC input; BPP output; regen output
function [APP, BPP, regen]= fcn(a, b, v, SOC)
    speed = v;
    if speed < 5
        regen = 0;
    elseif speed >= 25
        regen = 0.95;
    else
        regen = ((0.95/20)*speed)-0.2375;
    end

    APP = a + b*regen;
    BPP = (1-regen)*b;

== matlab function P4_car/Longitudinal Dynamics Body Frame/Electric Motor Drive/EM/MATLAB Function ==
  data: Tm input; I_bus output; Wm input; Effm input; V_bus input
function I_bus = fcn(Tm, Wm, Effm, V_bus)
    Pm = Tm*Wm;
    sgn_m = Pm / (abs(Pm+0.001));
    Pe = Pm * (Effm^sgn_m);
    
    I_bus = Pe/V_bus;
